simulink model "RizzoRezEq"  (Simulink 7.5)
settings: Solver=ode45  StartTime=0.0  StopTime=10.0  RelTol=1e-3
values from neighbouring files (symbols this model uses):
  Bc = 0    [TFconfirm.m]    (also in Torsonal_Model_Constants.m = 0.01)
  Ja = Ja+JL    (= 0.0056)    [TFconfirm.m]
  JL = 0.0033    [TFconfirm.m]    (also in Torsonal_Model_Constants.m)
  Kc = 0    [TFconfirm.m]
  ki = 0.2    [PlotRizzo.m]    (also in RizzoRezEqBode.m = 0.02; TFconfirm.m)
  Kt = 6.046    [PlotRizzo.m]    (also in RizzoRezEqBode.m; TFconfirm.m)
  kv = 20    [PlotRizzo.m]    (also in RizzoRezEqBode.m; TFconfirm.m)
  L = 0.842    [PlotRizzo.m]    (also in RizzoRezEqBode.m; TFconfirm.m)
  Ra = 0.38    [PlotRizzo.m]    (also in RizzoRezEqBode.m; TFconfirm.m)
settings Model: Creator=geovana  LastModifiedBy=geovana

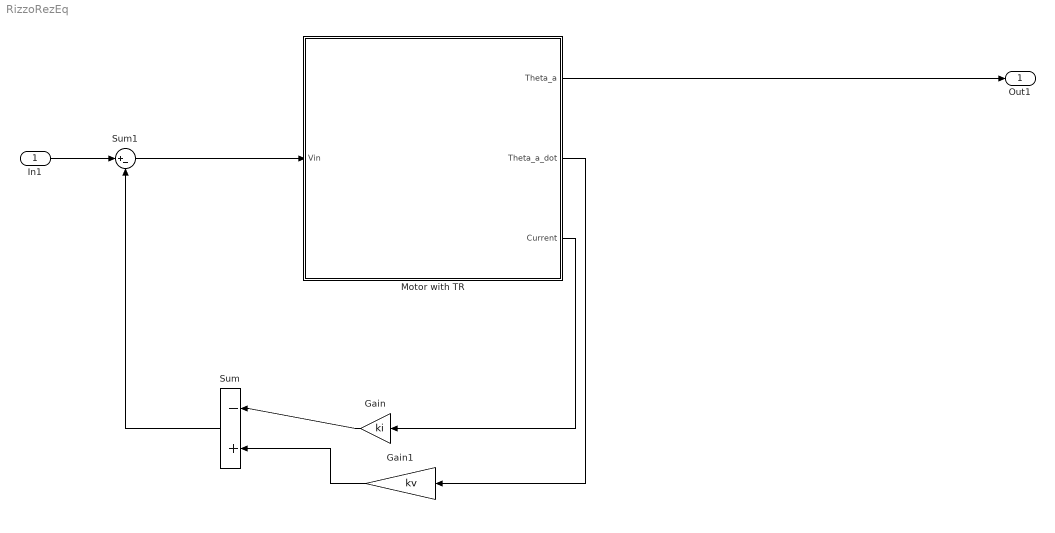
== system RizzoRezEq ==
  In1 : Inport  OutDataType=fixdt(1, 16)  OutScaling=2^0
  Gain : Gain  Gain=ki  ParameterDataType=fixdt(1, 16)  ParameterScaling=2^0  OutDataType=fixdt(1, 16)  OutScaling=2^0
  Gain1 : Gain  Gain=kv  ParameterDataType=fixdt(1, 16)  ParameterScaling=2^0  OutDataType=fixdt(1, 16)  OutScaling=2^0
  Motor with TR : Subsystem
  Sum : Sum  Inputs=|-+  OutDataType=fixdt(1, 16)  OutScaling=2^0
  Sum1 : Sum  Inputs=|+-  OutDataType=fixdt(1, 16)  OutScaling=2^0
  Out1 : Outport  OutDataType=fixdt(1, 16)  OutScaling=2^0
  wires:
  Motor with TR/1(Theta_a) -> Out1/1
  In1/1 -> Sum1/1
  Sum1/1 -> Motor with TR/1(Vin)
  Sum/1 -> Sum1/2
  Gain1/1 -> Sum/2
  Gain/1 -> Sum/1
  Motor with TR/3(Current) -> Gain/1
  Motor with TR/2(Theta_a_dot) -> Gain1/1

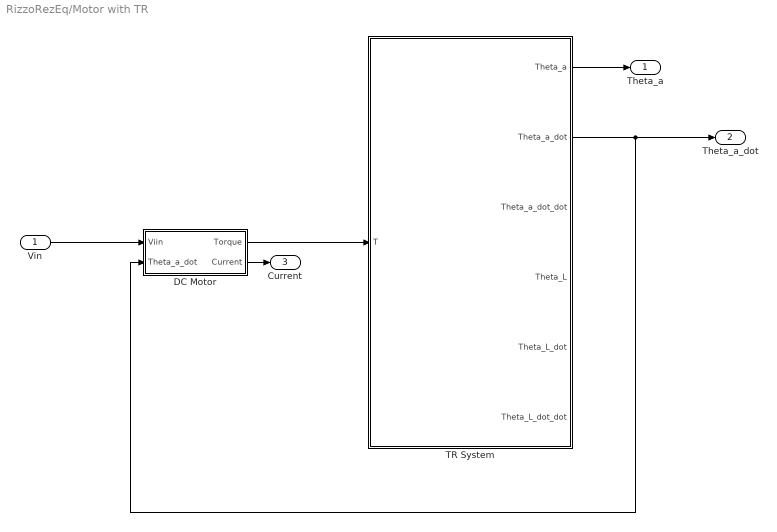
== system RizzoRezEq/Motor with TR ==
  Vin : Inport  OutDataType=fixdt(1, 16)  OutScaling=2^0
  DC Motor : Subsystem
  TR System : Subsystem
  Theta_a : Outport  OutDataType=fixdt(1, 16)  OutScaling=2^0
  Theta_a_dot : Outport  Port=2  OutDataType=fixdt(1, 16)  OutScaling=2^0
  Current : Outport  Port=3
  wires:
  DC Motor/1(Torque) -> TR System/1(T)
  TR System/2(Theta_a_dot) -> DC Motor/2(Theta_a_dot), Theta_a_dot/1
  Vin/1 -> DC Motor/1(Viin)
  TR System/1(Theta_a) -> Theta_a/1
  DC Motor/2(Current) -> Current/1

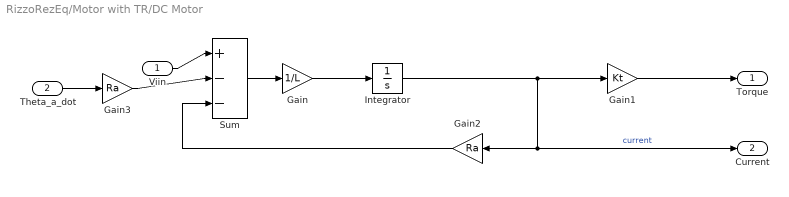
== system RizzoRezEq/Motor with TR/DC Motor ==
  Viin : Inport  OutDataType=fixdt(1, 16)  OutScaling=2^0
  Theta_a_dot : Inport  Port=2  OutDataType=fixdt(1, 16)  OutScaling=2^0
  Gain : Gain  Gain=1/L  ParameterDataType=fixdt(1, 16)  ParameterScaling=2^0  OutDataType=fixdt(1, 16)  OutScaling=2^0
  Gain1 : Gain  Gain=Kt  ParameterDataType=fixdt(1, 16)  ParameterScaling=2^0  OutDataType=fixdt(1, 16)  OutScaling=2^0
  Gain2 : Gain  Gain=Ra  ParameterDataType=fixdt(1, 16)  ParameterScaling=2^0  OutDataType=fixdt(1, 16)  OutScaling=2^0
  Gain3 : Gain  Gain=Ra  ParameterDataType=fixdt(1, 16)  ParameterScaling=2^0  OutDataType=fixdt(1, 16)  OutScaling=2^0
  Integrator : Integrator
  Sum : Sum  Inputs=|+--  OutDataType=fixdt(1, 16)  OutScaling=2^0
  Torque : Outport  OutDataType=fixdt(1, 16)  OutScaling=2^0
  Current : Outport  Port=2  OutDataType=fixdt(1, 16)  OutScaling=2^0
  wires:
  Viin/1 -> Sum/1
  Sum/1 -> Gain/1
  Gain/1 -> Integrator/1
  Integrator/1 -> Gain1/1, Current/1, Gain2/1  "current"
  Gain1/1 -> Torque/1
  Gain2/1 -> Sum/3
  Theta_a_dot/1 -> Gain3/1
  Gain3/1 -> Sum/2

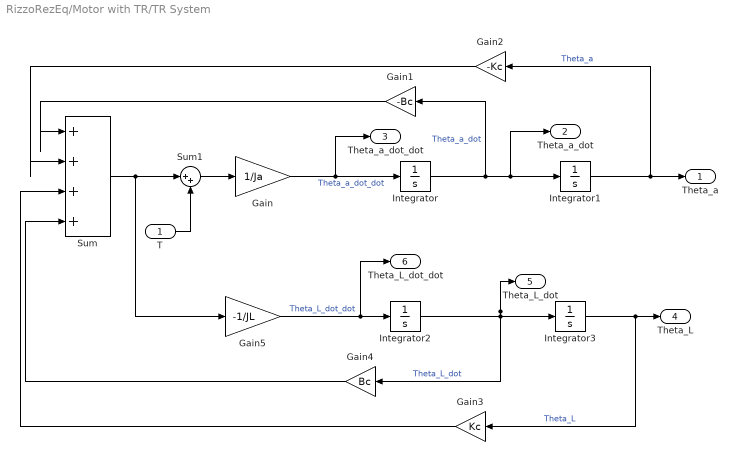
== system RizzoRezEq/Motor with TR/TR System ==
  T : Inport  OutDataType=sfix(16)  OutScaling=2^0
  Gain : Gain  Gain=1/Ja  ParameterDataType=sfix(16)  ParameterScaling=2^0  OutDataType=sfix(16)  OutScaling=2^0
  Gain1 : Gain  Gain=-Bc  ParameterDataType=sfix(16)  ParameterScaling=2^0  OutDataType=sfix(16)  OutScaling=2^0
  Gain2 : Gain  Gain=-Kc  ParameterDataType=sfix(16)  ParameterScaling=2^0  OutDataType=sfix(16)  OutScaling=2^0
  Gain3 : Gain  Gain=Kc  ParameterDataType=sfix(16)  ParameterScaling=2^0  OutDataType=sfix(16)  OutScaling=2^0
  Gain4 : Gain  Gain=Bc  ParameterDataType=sfix(16)  ParameterScaling=2^0  OutDataType=sfix(16)  OutScaling=2^0
  Gain5 : Gain  Gain=-1/JL  ParameterDataType=sfix(16)  ParameterScaling=2^0  OutDataType=sfix(16)  OutScaling=2^0
  Integrator{,1..3} (4 alike) : Integrator
  Sum : Sum  Inputs=|++++  OutDataType=sfix(16)  OutScaling=2^0
  Sum1 : Sum  Inputs=|++  OutDataType=sfix(16)  OutScaling=2^0
  Theta_a : Outport  OutDataType=sfix(16)  OutScaling=2^0
  Theta_a_dot : Outport  Port=2  OutDataType=sfix(16)  OutScaling=2^0
  Theta_a_dot_dot : Outport  Port=3  OutDataType=sfix(16)  OutScaling=2^0
  Theta_L : Outport  Port=4  OutDataType=sfix(16)  OutScaling=2^0
  Theta_L_dot : Outport  Port=5  OutDataType=sfix(16)  OutScaling=2^0
  Theta_L_dot_dot : Outport  Port=6  OutDataType=sfix(16)  OutScaling=2^0
  wires:
  Sum/1 -> Gain5/1, Sum1/1
  Integrator/1 -> Gain1/1, Integrator1/1, Theta_a_dot/1  "Theta_a_dot"
  Integrator1/1 -> Gain2/1, Theta_a/1  "Theta_a"
  Gain1/1 -> Sum/1
  Gain2/1 -> Sum/2
  Gain/1 -> Integrator/1, Theta_a_dot_dot/1  "Theta_a_dot_dot"
  Integrator2/1 -> Integrator3/1, Gain4/1, Theta_L_dot/1  "Theta_L_dot"
  Gain5/1 -> Integrator2/1, Theta_L_dot_dot/1  "Theta_L_dot_dot"
  Sum1/1 -> Gain/1
  T/1 -> Sum1/2
  Integrator3/1 -> Theta_L/1, Gain3/1  "Theta_L"
  Gain3/1 -> Sum/3
  Gain4/1 -> Sum/4
